simulink library "inp"  (R2021b)
settings: Solver=VariableStepAuto  StartTime=0.0  StopTime=10.0  RelTol=1e-3
undefined symbols (not defined in the file): C_TASK_5MS_S, FALSE, KINP_AcoreReadyToSlp_flg_ovrdflg, KINP_AcoreReadyToSlp_flg_ovrdval, KINP_AllowMovThd_OTA_enum_ovrdflg, KINP_AllowMovThd_OTA_enum_ovrdval, KINP_APSAngleTarget_Deg_ovrdflg, KINP_APSAngleTarget_Deg_ovrdval, KINP_APSDecReq_mps2_ovrdflg, KINP_APSDecReq_mps2_ovrdval, KINP_APSDecReqA_flg_ovrdflg, KINP_APSDecReqA_flg_ovrdval, KINP_APSDFLL_cm_ovrdflg, KINP_APSDFLL_cm_ovrdval, KINP_APSDFLR_cm_ovrdflg, KINP_APSDFLR_cm_ovrdval, KINP_APSDRLL_cm_ovrdflg, KINP_APSDRLL_cm_ovrdval, KINP_APSDRLR_cm_ovrdflg, KINP_APSDRLR_cm_ovrdval, KINP_APSExitCondition_enum_ovrdflg, KINP_APSExitCondition_enum_ovrdval, KINP_APSHWVer_enum_ovrdflg, KINP_APSHWVer_enum_ovrdval, KINP_APSProgressPCT_pct_ovrdflg, KINP_APSProgressPCT_pct_ovrdval, KINP_APSReq_enum_ovrdflg, KINP_APSReq_enum_ovrdval, KINP_APSRQDisplay_enum_ovrdflg, KINP_APSRQDisplay_enum_ovrdval, KINP_APSRqEPASCtrl_flg_ovrdflg, KINP_APSRqEPASCtrl_flg_ovrdval, KINP_APSShiftPosnReq_enum_ovrdval, KINP_APSShiftPosnReq_enum_ovrflg, KINP_APSSpeedCMD_kph_ovrdval, KINP_APSSpeedCMD_kph_ovrflg, KINP_APSStaSystem_enum_ovrdflg, KINP_APSStaSystem_enum_ovrdval, KINP_APSSWVer_enum_ovrdflg, KINP_APSSWVer_enum_ovrdval, KINP_APSVMCReqA_flg_ovrdval, KINP_APSVMCReqA_flg_ovrflg, KINP_APSVRqEPASCtrl_flg_ovrdflg, KINP_APSVRqEPASCtrl_flg_ovrdval, KINP_AuxBattVolmV_mV_ovrdflg, KINP_AuxBattVolmV_mV_ovrdval, KINP_CAASSta_enum_ovrdflg, KINP_CAASSta_enum_ovrdval, KINP_CAASVMCReqA_flg_ovrdval, KINP_CAASVMCReqA_flg_ovrflg, KINP_Chime_enum_ovrdflg, KINP_Chime_enum_ovrdval, KINP_ClearDTCcmd_flg_ovrdflg, KINP_ClearDTCcmd_flg_ovrdval, KINP_EvccAplusPwrUpReq_flg_ovrdflg, KINP_EvccAplusPwrUpReq_flg_ovrdval, KINP_LFID_raw_ovrdval, KINP_LFID_raw_ovrflg, KINP_LRID_raw_ovrdval, KINP_MemOffsetAccX_raw16_ovrdflg ... (+118)
libraries: FVT_lib x942, hcu_lib x1
(part 24 of 31)

== system inp/INP/CAN4/SignalCheck/ZONE_DR_VCU ==
  BHAL_outputs : Inport
  inp_CanValid_bus : Inport  Port=2
  BlowerErr : FVT_lib/inp/can_signal_template  SystemSampleTime=-1  VariantActivationTime=update diagram  Latency=0  AutoFrameSizeCalculation=off
      link override defval: Value=KINP_BlowerErr_enum_defval
      link override ovrdflg: Value=KINP_BlowerErr_enum_ovrdflg
      link override ovrdval: Value=KINP_BlowerErr_enum_ovrdval
  DrPMMLVOutPErrLmp : FVT_lib/inp/can_signal_template  SystemSampleTime=-1  VariantActivationTime=update diagram  Latency=0  AutoFrameSizeCalculation=off
      link override defval: Value=KINP_DrPMMLVOutPErrLmp_flg_defval
      link override ovrdflg: Value=KINP_DrPMMLVOutPErrLmp_flg_ovrdflg
      link override ovrdval: Value=KINP_DrPMMLVOutPErrLmp_flg_ovrdval
  DrPMMSysErrLmp : FVT_lib/inp/can_signal_template  SystemSampleTime=-1  VariantActivationTime=update diagram  Latency=0  AutoFrameSizeCalculation=off
      link override defval: Value=KINP_DrPMMSysErrLmp_flg_defval
      link override ovrdflg: Value=KINP_DrPMMSysErrLmp_flg_ovrdflg
      link override ovrdval: Value=KINP_DrPMMSysErrLmp_flg_ovrdval
  DrSCPSysErrLmp : FVT_lib/inp/can_signal_template  SystemSampleTime=-1  VariantActivationTime=update diagram  Latency=0  AutoFrameSizeCalculation=off
      link override defval: Value=KINP_DrSCPSysErrLmp_flg_defval
      link override ovrdflg: Value=KINP_DrSCPSysErrLmp_flg_ovrdflg
      link override ovrdval: Value=KINP_DrSCPSysErrLmp_flg_ovrdval
  DrStdAErrSta : FVT_lib/inp/can_signal_template  SystemSampleTime=-1  VariantActivationTime=update diagram  Latency=0  AutoFrameSizeCalculation=off
      link override defval: Value=KINP_DrStdAErrSta_flg_defval
      link override ovrdflg: Value=KINP_DrStdAErrSta_flg_ovrdflg
      link override ovrdval: Value=KINP_DrStdAErrSta_flg_ovrdval
  SolarL : FVT_lib/inp/can_signal_template  SystemSampleTime=-1  VariantActivationTime=update diagram  Latency=0  AutoFrameSizeCalculation=off
      link override defval: Value=KINP_SolarL_W_defval
      link override ovrdflg: Value=KINP_SolarL_W_ovrdflg
      link override ovrdval: Value=KINP_SolarL_W_ovrdval
  SolarLErr : FVT_lib/inp/can_signal_template  SystemSampleTime=-1  VariantActivationTime=update diagram  Latency=0  AutoFrameSizeCalculation=off
      link override defval: Value=KINP_SolarLErr_enum_defval
      link override ovrdflg: Value=KINP_SolarLErr_enum_ovrdflg
      link override ovrdval: Value=KINP_SolarLErr_enum_ovrdval
  SolarR : FVT_lib/inp/can_signal_template  SystemSampleTime=-1  VariantActivationTime=update diagram  Latency=0  AutoFrameSizeCalculation=off
      link override defval: Value=KINP_SolarR_W_defval
      link override ovrdflg: Value=KINP_SolarR_W_ovrdflg
      link override ovrdval: Value=KINP_SolarR_W_ovrdval
  SolarRErr : FVT_lib/inp/can_signal_template  SystemSampleTime=-1  VariantActivationTime=update diagram  Latency=0  AutoFrameSizeCalculation=off
      link override defval: Value=KINP_SolarRErr_enum_defval
      link override ovrdflg: Value=KINP_SolarRErr_enum_ovrdflg
      link override ovrdval: Value=KINP_SolarRErr_enum_ovrdval
  TFaceL : FVT_lib/inp/can_signal_template  SystemSampleTime=-1  VariantActivationTime=update diagram  Latency=0  AutoFrameSizeCalculation=off
      link override defval: Value=KINP_TFaceL_C_defval
      link override ovrdflg: Value=KINP_TFaceL_C_ovrdflg
      link override ovrdval: Value=KINP_TFaceL_C_ovrdval
  TFaceLErr : FVT_lib/inp/can_signal_template  SystemSampleTime=-1  VariantActivationTime=update diagram  Latency=0  AutoFrameSizeCalculation=off
      link override defval: Value=KINP_TFaceLErr_enum_defval
      link override ovrdflg: Value=KINP_TFaceLErr_enum_ovrdflg
      link override ovrdval: Value=KINP_TFaceLErr_enum_ovrdval
  TFaceR : FVT_lib/inp/can_signal_template  SystemSampleTime=-1  VariantActivationTime=update diagram  Latency=0  AutoFrameSizeCalculation=off
      link override defval: Value=KINP_TFaceR_C_defval
      link override ovrdflg: Value=KINP_TFaceR_C_ovrdflg
      link override ovrdval: Value=KINP_TFaceR_C_ovrdval
  TFaceRErr : FVT_lib/inp/can_signal_template  SystemSampleTime=-1  VariantActivationTime=update diagram  Latency=0  AutoFrameSizeCalculation=off
      link override defval: Value=KINP_TFaceRErr_enum_defval
      link override ovrdflg: Value=KINP_TFaceRErr_enum_ovrdflg
      link override ovrdval: Value=KINP_TFaceRErr_enum_ovrdval
  TFaceRr : FVT_lib/inp/can_signal_template  SystemSampleTime=-1  VariantActivationTime=update diagram  Latency=0  AutoFrameSizeCalculation=off
      link override defval: Value=KINP_TFaceRr_C_defval
      link override ovrdflg: Value=KINP_TFaceRr_C_ovrdflg
      link override ovrdval: Value=KINP_TFaceRr_C_ovrdval
  TFaceRrErr : FVT_lib/inp/can_signal_template  SystemSampleTime=-1  VariantActivationTime=update diagram  Latency=0  AutoFrameSizeCalculation=off
      link override defval: Value=KINP_TFaceRrErr_enum_defval
      link override ovrdflg: Value=KINP_TFaceRrErr_enum_ovrdflg
      link override ovrdval: Value=KINP_TFaceRrErr_enum_ovrdval
  TFootL : FVT_lib/inp/can_signal_template  SystemSampleTime=-1  VariantActivationTime=update diagram  Latency=0  AutoFrameSizeCalculation=off
      link override defval: Value=KINP_TFootL_C_defval
      link override ovrdflg: Value=KINP_TFootL_C_ovrdflg
      link override ovrdval: Value=KINP_TFootL_C_ovrdval
  TFootLErr : FVT_lib/inp/can_signal_template  SystemSampleTime=-1  VariantActivationTime=update diagram  Latency=0  AutoFrameSizeCalculation=off
      link override defval: Value=KINP_TFootLErr_enum_defval
      link override ovrdflg: Value=KINP_TFootLErr_enum_ovrdflg
      link override ovrdval: Value=KINP_TFootLErr_enum_ovrdval
  TFootR : FVT_lib/inp/can_signal_template  SystemSampleTime=-1  VariantActivationTime=update diagram  Latency=0  AutoFrameSizeCalculation=off
      link override defval: Value=KINP_TFootR_C_defval
      link override ovrdflg: Value=KINP_TFootR_C_ovrdflg
      link override ovrdval: Value=KINP_TFootR_C_ovrdval
  TFootRErr : FVT_lib/inp/can_signal_template  SystemSampleTime=-1  VariantActivationTime=update diagram  Latency=0  AutoFrameSizeCalculation=off
      link override defval: Value=KINP_TFootRErr_enum_defval
      link override ovrdflg: Value=KINP_TFootRErr_enum_ovrdflg
      link override ovrdval: Value=KINP_TFootRErr_enum_ovrdval
  TFootRr : FVT_lib/inp/can_signal_template  SystemSampleTime=-1  VariantActivationTime=update diagram  Latency=0  AutoFrameSizeCalculation=off
      link override defval: Value=KINP_TFootRr_C_defval
      link override ovrdflg: Value=KINP_TFootRr_C_ovrdflg
      link override ovrdval: Value=KINP_TFootRr_C_ovrdval
  TFootRrErr : FVT_lib/inp/can_signal_template  SystemSampleTime=-1  VariantActivationTime=update diagram  Latency=0  AutoFrameSizeCalculation=off
      link override defval: Value=KINP_TFootRrErr_enum_defval
      link override ovrdflg: Value=KINP_TFootRrErr_enum_ovrdflg
      link override ovrdval: Value=KINP_TFootRrErr_enum_ovrdval
  Terminator_{1..26} (26 alike) : Terminator
  Tevap : FVT_lib/inp/can_signal_template  SystemSampleTime=-1  VariantActivationTime=update diagram  Latency=0  AutoFrameSizeCalculation=off
      link override defval: Value=KINP_Tevap_C_defval
      link override ovrdflg: Value=KINP_Tevap_C_ovrdflg
      link override ovrdval: Value=KINP_Tevap_C_ovrdval
  TevapErr : FVT_lib/inp/can_signal_template  SystemSampleTime=-1  VariantActivationTime=update diagram  Latency=0  AutoFrameSizeCalculation=off
      link override defval: Value=KINP_TevapErr_enum_defval
      link override ovrdflg: Value=KINP_TevapErr_enum_ovrdflg
      link override ovrdval: Value=KINP_TevapErr_enum_ovrdval
  Tincar : FVT_lib/inp/can_signal_template  SystemSampleTime=-1  VariantActivationTime=update diagram  Latency=0  AutoFrameSizeCalculation=off
      link override defval: Value=KINP_Tincar_C_defval
      link override ovrdflg: Value=KINP_Tincar_C_ovrdflg
      link override ovrdval: Value=KINP_Tincar_C_ovrdval
  TincarErr : FVT_lib/inp/can_signal_template  SystemSampleTime=-1  VariantActivationTime=update diagram  Latency=0  AutoFrameSizeCalculation=off
      link override defval: Value=KINP_TincarErr_enum_defval
      link override ovrdflg: Value=KINP_TincarErr_enum_ovrdflg
      link override ovrdval: Value=KINP_TincarErr_enum_ovrdval
  True_VHAL_BlowerErr_enum : Constant  Value=TRUE  OutDataTypeStr=boolean
  True_VHAL_DrPMMLVOutPErrLmp_flg : Constant  Value=TRUE  OutDataTypeStr=boolean
  True_VHAL_DrPMMSysErrLmp_flg : Constant  Value=TRUE  OutDataTypeStr=boolean
  True_VHAL_DrSCPSysErrLmp_flg : Constant  Value=TRUE  OutDataTypeStr=boolean
  True_VHAL_DrStdAErrSta_flg : Constant  Value=TRUE  OutDataTypeStr=boolean
  True_VHAL_SolarLErr_enum : Constant  Value=TRUE  OutDataTypeStr=boolean
  True_VHAL_SolarL_W : Constant  Value=TRUE  OutDataTypeStr=boolean
  True_VHAL_SolarRErr_enum : Constant  Value=TRUE  OutDataTypeStr=boolean
  True_VHAL_SolarR_W : Constant  Value=TRUE  OutDataTypeStr=boolean
  True_VHAL_TFaceLErr_enum : Constant  Value=TRUE  OutDataTypeStr=boolean
  True_VHAL_TFaceL_C : Constant  Value=TRUE  OutDataTypeStr=boolean
  True_VHAL_TFaceRErr_enum : Constant  Value=TRUE  OutDataTypeStr=boolean
  True_VHAL_TFaceR_C : Constant  Value=TRUE  OutDataTypeStr=boolean
  True_VHAL_TFaceRrErr_enum : Constant  Value=TRUE  OutDataTypeStr=boolean
  True_VHAL_TFaceRr_C : Constant  Value=TRUE  OutDataTypeStr=boolean
  True_VHAL_TFootLErr_enum : Constant  Value=TRUE  OutDataTypeStr=boolean
  True_VHAL_TFootL_C : Constant  Value=TRUE  OutDataTypeStr=boolean
  True_VHAL_TFootRErr_enum : Constant  Value=TRUE  OutDataTypeStr=boolean
  True_VHAL_TFootR_C : Constant  Value=TRUE  OutDataTypeStr=boolean
  True_VHAL_TFootRrErr_enum : Constant  Value=TRUE  OutDataTypeStr=boolean
  True_VHAL_TFootRr_C : Constant  Value=TRUE  OutDataTypeStr=boolean
  True_VHAL_TevapErr_enum : Constant  Value=TRUE  OutDataTypeStr=boolean
  True_VHAL_Tevap_C : Constant  Value=TRUE  OutDataTypeStr=boolean
  True_VHAL_TincarErr_enum : Constant  Value=TRUE  OutDataTypeStr=boolean
  True_VHAL_Tincar_C : Constant  Value=TRUE  OutDataTypeStr=boolean
  True_VHAL_ZoneDrMalfunLevel_enum : Constant  Value=TRUE  OutDataTypeStr=boolean
  ZoneDrMalfunLevel : FVT_lib/inp/can_signal_template  SystemSampleTime=-1  VariantActivationTime=update diagram  Latency=0  AutoFrameSizeCalculation=off
      link override defval: Value=KINP_ZoneDrMalfunLevel_enum_defval
      link override ovrdflg: Value=KINP_ZoneDrMalfunLevel_enum_ovrdflg
      link override ovrdval: Value=KINP_ZoneDrMalfunLevel_enum_ovrdval
  slr1_{1..26} (26 alike) : BusSelector  OutputSignals=VINP_CANMsgValidZONEDRVCU_flg
  slr_VHAL_BlowerErr_enum : BusSelector  OutputSignals=VHAL_BlowerErr_enum
  slr_VHAL_DrPMMLVOutPErrLmp_flg : BusSelector  OutputSignals=VHAL_DrPMMLVOutPErrLmp_flg
  slr_VHAL_DrPMMSysErrLmp_flg : BusSelector  OutputSignals=VHAL_DrPMMSysErrLmp_flg
  slr_VHAL_DrSCPSysErrLmp_flg : BusSelector  OutputSignals=VHAL_DrSCPSysErrLmp_flg
  slr_VHAL_DrStdAErrSta_flg : BusSelector  OutputSignals=VHAL_DrStdAErrSta_flg
  slr_VHAL_SolarLErr_enum : BusSelector  OutputSignals=VHAL_SolarLErr_enum
  slr_VHAL_SolarL_W : BusSelector  OutputSignals=VHAL_SolarL_W
  slr_VHAL_SolarRErr_enum : BusSelector  OutputSignals=VHAL_SolarRErr_enum
  slr_VHAL_SolarR_W : BusSelector  OutputSignals=VHAL_SolarR_W
  slr_VHAL_TFaceLErr_enum : BusSelector  OutputSignals=VHAL_TFaceLErr_enum
  slr_VHAL_TFaceL_C : BusSelector  OutputSignals=VHAL_TFaceL_C
  slr_VHAL_TFaceRErr_enum : BusSelector  OutputSignals=VHAL_TFaceRErr_enum
  slr_VHAL_TFaceR_C : BusSelector  OutputSignals=VHAL_TFaceR_C
  slr_VHAL_TFaceRrErr_enum : BusSelector  OutputSignals=VHAL_TFaceRrErr_enum
  slr_VHAL_TFaceRr_C : BusSelector  OutputSignals=VHAL_TFaceRr_C
  slr_VHAL_TFootLErr_enum : BusSelector  OutputSignals=VHAL_TFootLErr_enum
  slr_VHAL_TFootL_C : BusSelector  OutputSignals=VHAL_TFootL_C
  slr_VHAL_TFootRErr_enum : BusSelector  OutputSignals=VHAL_TFootRErr_enum
  slr_VHAL_TFootR_C : BusSelector  OutputSignals=VHAL_TFootR_C
  slr_VHAL_TFootRrErr_enum : BusSelector  OutputSignals=VHAL_TFootRrErr_enum
  slr_VHAL_TFootRr_C : BusSelector  OutputSignals=VHAL_TFootRr_C
  slr_VHAL_TevapErr_enum : BusSelector  OutputSignals=VHAL_TevapErr_enum
  slr_VHAL_Tevap_C : BusSelector  OutputSignals=VHAL_Tevap_C
  slr_VHAL_TincarErr_enum : BusSelector  OutputSignals=VHAL_TincarErr_enum
  slr_VHAL_Tincar_C : BusSelector  OutputSignals=VHAL_Tincar_C
  slr_VHAL_ZoneDrMalfunLevel_enum : BusSelector  OutputSignals=VHAL_ZoneDrMalfunLevel_enum
  VINP_BlowerErr_enum : Outport
  VINP_DrPMMLVOutPErrLmp_flg : Outport  Port=2
  VINP_DrPMMSysErrLmp_flg : Outport  Port=3
  VINP_DrSCPSysErrLmp_flg : Outport  Port=4
  VINP_DrStdAErrSta_flg : Outport  Port=5
  VINP_SolarL_W : Outport  Port=6
  VINP_SolarLErr_enum : Outport  Port=7
  VINP_SolarR_W : Outport  Port=8
  VINP_SolarRErr_enum : Outport  Port=9
  VINP_TFaceL_C : Outport  Port=10
  VINP_TFaceLErr_enum : Outport  Port=11
  VINP_TFaceR_C : Outport  Port=12
  VINP_TFaceRErr_enum : Outport  Port=13
  VINP_TFaceRr_C : Outport  Port=14
  VINP_TFaceRrErr_enum : Outport  Port=15
  VINP_TFootL_C : Outport  Port=16
  VINP_TFootLErr_enum : Outport  Port=17
  VINP_TFootR_C : Outport  Port=18
  VINP_TFootRErr_enum : Outport  Port=19
  VINP_TFootRr_C : Outport  Port=20
  VINP_TFootRrErr_enum : Outport  Port=21
  VINP_Tevap_C : Outport  Port=22
  VINP_TevapErr_enum : Outport  Port=23
  VINP_Tincar_C : Outport  Port=24
  VINP_TincarErr_enum : Outport  Port=25
  VINP_ZoneDrMalfunLevel_enum : Outport  Port=26
  wires:
  BHAL_outputs/1 -> [BHAL_outputs]
  inp_CanValid_bus/1 -> [inp_CanValid_bus]
  [BHAL_outputs] -> slr_VHAL_BlowerErr_enum/1
  slr_VHAL_BlowerErr_enum/1 -> BlowerErr/1  "<VHAL_BlowerErr_enum>"
  True_VHAL_BlowerErr_enum/1 -> BlowerErr/2
  [inp_CanValid_bus] -> slr1_1/1
  slr1_1/1 -> BlowerErr/3  "<VINP_CANMsgValidZONEDRVCU_flg>"
  BlowerErr/1 -> VINP_BlowerErr_enum/1  "VINP_BlowerErr_enum"
  BlowerErr/2 -> Terminator_1/1
  [BHAL_outputs] -> slr_VHAL_DrPMMLVOutPErrLmp_flg/1
  slr_VHAL_DrPMMLVOutPErrLmp_flg/1 -> DrPMMLVOutPErrLmp/1  "<VHAL_DrPMMLVOutPErrLmp_flg>"
  True_VHAL_DrPMMLVOutPErrLmp_flg/1 -> DrPMMLVOutPErrLmp/2
  [inp_CanValid_bus] -> slr1_2/1
  slr1_2/1 -> DrPMMLVOutPErrLmp/3  "<VINP_CANMsgValidZONEDRVCU_flg>"
  DrPMMLVOutPErrLmp/1 -> VINP_DrPMMLVOutPErrLmp_flg/1  "VINP_DrPMMLVOutPErrLmp_flg"
  DrPMMLVOutPErrLmp/2 -> Terminator_2/1
  [BHAL_outputs] -> slr_VHAL_DrPMMSysErrLmp_flg/1
  slr_VHAL_DrPMMSysErrLmp_flg/1 -> DrPMMSysErrLmp/1  "<VHAL_DrPMMSysErrLmp_flg>"
  True_VHAL_DrPMMSysErrLmp_flg/1 -> DrPMMSysErrLmp/2
  [inp_CanValid_bus] -> slr1_3/1
  slr1_3/1 -> DrPMMSysErrLmp/3  "<VINP_CANMsgValidZONEDRVCU_flg>"
  DrPMMSysErrLmp/1 -> VINP_DrPMMSysErrLmp_flg/1  "VINP_DrPMMSysErrLmp_flg"
  DrPMMSysErrLmp/2 -> Terminator_3/1
  [BHAL_outputs] -> slr_VHAL_DrSCPSysErrLmp_flg/1
  slr_VHAL_DrSCPSysErrLmp_flg/1 -> DrSCPSysErrLmp/1  "<VHAL_DrSCPSysErrLmp_flg>"
  True_VHAL_DrSCPSysErrLmp_flg/1 -> DrSCPSysErrLmp/2
  [inp_CanValid_bus] -> slr1_4/1
  slr1_4/1 -> DrSCPSysErrLmp/3  "<VINP_CANMsgValidZONEDRVCU_flg>"
  DrSCPSysErrLmp/1 -> VINP_DrSCPSysErrLmp_flg/1  "VINP_DrSCPSysErrLmp_flg"
  DrSCPSysErrLmp/2 -> Terminator_4/1
  [BHAL_outputs] -> slr_VHAL_DrStdAErrSta_flg/1
  slr_VHAL_DrStdAErrSta_flg/1 -> DrStdAErrSta/1  "<VHAL_DrStdAErrSta_flg>"
  True_VHAL_DrStdAErrSta_flg/1 -> DrStdAErrSta/2
  [inp_CanValid_bus] -> slr1_5/1
  slr1_5/1 -> DrStdAErrSta/3  "<VINP_CANMsgValidZONEDRVCU_flg>"
  DrStdAErrSta/1 -> VINP_DrStdAErrSta_flg/1  "VINP_DrStdAErrSta_flg"
  DrStdAErrSta/2 -> Terminator_5/1
  [BHAL_outputs] -> slr_VHAL_SolarL_W/1
  slr_VHAL_SolarL_W/1 -> SolarL/1  "<VHAL_SolarL_W>"
  True_VHAL_SolarL_W/1 -> SolarL/2
  [inp_CanValid_bus] -> slr1_6/1
  slr1_6/1 -> SolarL/3  "<VINP_CANMsgValidZONEDRVCU_flg>"
  SolarL/1 -> VINP_SolarL_W/1  "VINP_SolarL_W"
  SolarL/2 -> Terminator_6/1
  [BHAL_outputs] -> slr_VHAL_SolarLErr_enum/1
  slr_VHAL_SolarLErr_enum/1 -> SolarLErr/1  "<VHAL_SolarLErr_enum>"
  True_VHAL_SolarLErr_enum/1 -> SolarLErr/2
  [inp_CanValid_bus] -> slr1_7/1
  slr1_7/1 -> SolarLErr/3  "<VINP_CANMsgValidZONEDRVCU_flg>"
  SolarLErr/1 -> VINP_SolarLErr_enum/1  "VINP_SolarLErr_enum"
  SolarLErr/2 -> Terminator_7/1
  [BHAL_outputs] -> slr_VHAL_SolarR_W/1
  slr_VHAL_SolarR_W/1 -> SolarR/1  "<VHAL_SolarR_W>"
  True_VHAL_SolarR_W/1 -> SolarR/2
  [inp_CanValid_bus] -> slr1_8/1
  slr1_8/1 -> SolarR/3  "<VINP_CANMsgValidZONEDRVCU_flg>"
  SolarR/1 -> VINP_SolarR_W/1  "VINP_SolarR_W"
  SolarR/2 -> Terminator_8/1
  [BHAL_outputs] -> slr_VHAL_SolarRErr_enum/1
  slr_VHAL_SolarRErr_enum/1 -> SolarRErr/1  "<VHAL_SolarRErr_enum>"
  True_VHAL_SolarRErr_enum/1 -> SolarRErr/2
  [inp_CanValid_bus] -> slr1_9/1
  slr1_9/1 -> SolarRErr/3  "<VINP_CANMsgValidZONEDRVCU_flg>"
  SolarRErr/1 -> VINP_SolarRErr_enum/1  "VINP_SolarRErr_enum"
  SolarRErr/2 -> Terminator_9/1
  [BHAL_outputs] -> slr_VHAL_TFaceL_C/1
  slr_VHAL_TFaceL_C/1 -> TFaceL/1  "<VHAL_TFaceL_C>"
  True_VHAL_TFaceL_C/1 -> TFaceL/2
  [inp_CanValid_bus] -> slr1_10/1
  slr1_10/1 -> TFaceL/3  "<VINP_CANMsgValidZONEDRVCU_flg>"
  TFaceL/1 -> VINP_TFaceL_C/1  "VINP_TFaceL_C"
  TFaceL/2 -> Terminator_10/1
  [BHAL_outputs] -> slr_VHAL_TFaceLErr_enum/1
  slr_VHAL_TFaceLErr_enum/1 -> TFaceLErr/1  "<VHAL_TFaceLErr_enum>"
  True_VHAL_TFaceLErr_enum/1 -> TFaceLErr/2
  [inp_CanValid_bus] -> slr1_11/1
  slr1_11/1 -> TFaceLErr/3  "<VINP_CANMsgValidZONEDRVCU_flg>"
  TFaceLErr/1 -> VINP_TFaceLErr_enum/1  "VINP_TFaceLErr_enum"
  TFaceLErr/2 -> Terminator_11/1
  [BHAL_outputs] -> slr_VHAL_TFaceR_C/1
  slr_VHAL_TFaceR_C/1 -> TFaceR/1  "<VHAL_TFaceR_C>"
  True_VHAL_TFaceR_C/1 -> TFaceR/2
  [inp_CanValid_bus] -> slr1_12/1
  slr1_12/1 -> TFaceR/3  "<VINP_CANMsgValidZONEDRVCU_flg>"
  TFaceR/1 -> VINP_TFaceR_C/1  "VINP_TFaceR_C"
  TFaceR/2 -> Terminator_12/1
  [BHAL_outputs] -> slr_VHAL_TFaceRErr_enum/1
  slr_VHAL_TFaceRErr_enum/1 -> TFaceRErr/1  "<VHAL_TFaceRErr_enum>"
  True_VHAL_TFaceRErr_enum/1 -> TFaceRErr/2
  [inp_CanValid_bus] -> slr1_13/1
  slr1_13/1 -> TFaceRErr/3  "<VINP_CANMsgValidZONEDRVCU_flg>"
  TFaceRErr/1 -> VINP_TFaceRErr_enum/1  "VINP_TFaceRErr_enum"
  TFaceRErr/2 -> Terminator_13/1
  [BHAL_outputs] -> slr_VHAL_TFaceRr_C/1
  slr_VHAL_TFaceRr_C/1 -> TFaceRr/1  "<VHAL_TFaceRr_C>"
  True_VHAL_TFaceRr_C/1 -> TFaceRr/2
  [inp_CanValid_bus] -> slr1_14/1
  slr1_14/1 -> TFaceRr/3  "<VINP_CANMsgValidZONEDRVCU_flg>"
  TFaceRr/1 -> VINP_TFaceRr_C/1  "VINP_TFaceRr_C"
  TFaceRr/2 -> Terminator_14/1
  [BHAL_outputs] -> slr_VHAL_TFaceRrErr_enum/1
  slr_VHAL_TFaceRrErr_enum/1 -> TFaceRrErr/1  "<VHAL_TFaceRrErr_enum>"
  True_VHAL_TFaceRrErr_enum/1 -> TFaceRrErr/2
  [inp_CanValid_bus] -> slr1_15/1
  slr1_15/1 -> TFaceRrErr/3  "<VINP_CANMsgValidZONEDRVCU_flg>"
  TFaceRrErr/1 -> VINP_TFaceRrErr_enum/1  "VINP_TFaceRrErr_enum"
  TFaceRrErr/2 -> Terminator_15/1
  [BHAL_outputs] -> slr_VHAL_TFootL_C/1
  slr_VHAL_TFootL_C/1 -> TFootL/1  "<VHAL_TFootL_C>"
  True_VHAL_TFootL_C/1 -> TFootL/2
  [inp_CanValid_bus] -> slr1_16/1
  slr1_16/1 -> TFootL/3  "<VINP_CANMsgValidZONEDRVCU_flg>"
  TFootL/1 -> VINP_TFootL_C/1  "VINP_TFootL_C"
  TFootL/2 -> Terminator_16/1
  [BHAL_outputs] -> slr_VHAL_TFootLErr_enum/1
  slr_VHAL_TFootLErr_enum/1 -> TFootLErr/1  "<VHAL_TFootLErr_enum>"
  True_VHAL_TFootLErr_enum/1 -> TFootLErr/2
  [inp_CanValid_bus] -> slr1_17/1
  slr1_17/1 -> TFootLErr/3  "<VINP_CANMsgValidZONEDRVCU_flg>"
  TFootLErr/1 -> VINP_TFootLErr_enum/1  "VINP_TFootLErr_enum"
  TFootLErr/2 -> Terminator_17/1
  [BHAL_outputs] -> slr_VHAL_TFootR_C/1
  slr_VHAL_TFootR_C/1 -> TFootR/1  "<VHAL_TFootR_C>"
  True_VHAL_TFootR_C/1 -> TFootR/2
  [inp_CanValid_bus] -> slr1_18/1
  slr1_18/1 -> TFootR/3  "<VINP_CANMsgValidZONEDRVCU_flg>"
  TFootR/1 -> VINP_TFootR_C/1  "VINP_TFootR_C"
  TFootR/2 -> Terminator_18/1
  [BHAL_outputs] -> slr_VHAL_TFootRErr_enum/1
  slr_VHAL_TFootRErr_enum/1 -> TFootRErr/1  "<VHAL_TFootRErr_enum>"
  True_VHAL_TFootRErr_enum/1 -> TFootRErr/2
  [inp_CanValid_bus] -> slr1_19/1
  slr1_19/1 -> TFootRErr/3  "<VINP_CANMsgValidZONEDRVCU_flg>"
  TFootRErr/1 -> VINP_TFootRErr_enum/1  "VINP_TFootRErr_enum"
  TFootRErr/2 -> Terminator_19/1
  [BHAL_outputs] -> slr_VHAL_TFootRr_C/1
  slr_VHAL_TFootRr_C/1 -> TFootRr/1  "<VHAL_TFootRr_C>"
  True_VHAL_TFootRr_C/1 -> TFootRr/2
  [inp_CanValid_bus] -> slr1_20/1
  slr1_20/1 -> TFootRr/3  "<VINP_CANMsgValidZONEDRVCU_flg>"
  TFootRr/1 -> VINP_TFootRr_C/1  "VINP_TFootRr_C"
  TFootRr/2 -> Terminator_20/1
  [BHAL_outputs] -> slr_VHAL_TFootRrErr_enum/1
  slr_VHAL_TFootRrErr_enum/1 -> TFootRrErr/1  "<VHAL_TFootRrErr_enum>"
  True_VHAL_TFootRrErr_enum/1 -> TFootRrErr/2
  [inp_CanValid_bus] -> slr1_21/1
  slr1_21/1 -> TFootRrErr/3  "<VINP_CANMsgValidZONEDRVCU_flg>"
  TFootRrErr/1 -> VINP_TFootRrErr_enum/1  "VINP_TFootRrErr_enum"
  TFootRrErr/2 -> Terminator_21/1
  [BHAL_outputs] -> slr_VHAL_Tevap_C/1
  slr_VHAL_Tevap_C/1 -> Tevap/1  "<VHAL_Tevap_C>"
  True_VHAL_Tevap_C/1 -> Tevap/2
  [inp_CanValid_bus] -> slr1_22/1
  slr1_22/1 -> Tevap/3  "<VINP_CANMsgValidZONEDRVCU_flg>"
  Tevap/1 -> VINP_Tevap_C/1  "VINP_Tevap_C"
  Tevap/2 -> Terminator_22/1
  [BHAL_outputs] -> slr_VHAL_TevapErr_enum/1
  slr_VHAL_TevapErr_enum/1 -> TevapErr/1  "<VHAL_TevapErr_enum>"
  True_VHAL_TevapErr_enum/1 -> TevapErr/2
  [inp_CanValid_bus] -> slr1_23/1
  slr1_23/1 -> TevapErr/3  "<VINP_CANMsgValidZONEDRVCU_flg>"
  TevapErr/1 -> VINP_TevapErr_enum/1  "VINP_TevapErr_enum"
  TevapErr/2 -> Terminator_23/1
  [BHAL_outputs] -> slr_VHAL_Tincar_C/1
  slr_VHAL_Tincar_C/1 -> Tincar/1  "<VHAL_Tincar_C>"
  True_VHAL_Tincar_C/1 -> Tincar/2
  [inp_CanValid_bus] -> slr1_24/1
  slr1_24/1 -> Tincar/3  "<VINP_CANMsgValidZONEDRVCU_flg>"
  Tincar/1 -> VINP_Tincar_C/1  "VINP_Tincar_C"
  Tincar/2 -> Terminator_24/1
  [BHAL_outputs] -> slr_VHAL_TincarErr_enum/1
  slr_VHAL_TincarErr_enum/1 -> TincarErr/1  "<VHAL_TincarErr_enum>"
  True_VHAL_TincarErr_enum/1 -> TincarErr/2
  [inp_CanValid_bus] -> slr1_25/1
  slr1_25/1 -> TincarErr/3  "<VINP_CANMsgValidZONEDRVCU_flg>"
  TincarErr/1 -> VINP_TincarErr_enum/1  "VINP_TincarErr_enum"
  TincarErr/2 -> Terminator_25/1
  [BHAL_outputs] -> slr_VHAL_ZoneDrMalfunLevel_enum/1
  slr_VHAL_ZoneDrMalfunLevel_enum/1 -> ZoneDrMalfunLevel/1  "<VHAL_ZoneDrMalfunLevel_enum>"
  True_VHAL_ZoneDrMalfunLevel_enum/1 -> ZoneDrMalfunLevel/2
  [inp_CanValid_bus] -> slr1_26/1
  slr1_26/1 -> ZoneDrMalfunLevel/3  "<VINP_CANMsgValidZONEDRVCU_flg>"
  ZoneDrMalfunLevel/1 -> VINP_ZoneDrMalfunLevel_enum/1  "VINP_ZoneDrMalfunLevel_enum"
  ZoneDrMalfunLevel/2 -> Terminator_26/1
